simulink model "csu_gmb_gimbal_motor_actuator_diag"  (R2015b)
settings: Solver=VariableStepAuto  StartTime=0.0  StopTime=10.0  RelTol=1e-3
values from neighbouring files (symbols this model uses):
  Bm = gim_motor_Bm    [csu_gmb_motor_prep.m]
  Jm = gim_motor_Jm    [csu_gmb_motor_prep.m]
  Ke = gim_motor_Ke    [csu_gmb_motor_prep.m]
  Kl = gim_motor_Kl    [csu_gmb_motor_prep.m]
  Kt = gim_motor_Kt    [csu_gmb_motor_prep.m]
  Lm = gim_motor_Lm    [csu_gmb_motor_prep.m]
  nb = gim_motor_nb    [csu_gmb_motor_prep.m]
  Rm = gim_motor_Rm    [csu_gmb_motor_prep.m]
undefined symbols (not defined in the file or in its folder): DiscIntNeverNeededParam
settings Model: Creator=jimkaidy  LastModifiedBy=jimkaidy

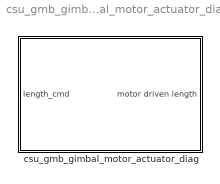
== system csu_gmb_gimbal_motor_actuator_diag ==
  csu_gmb_gimbal_motor_actuator_diag : Subsystem

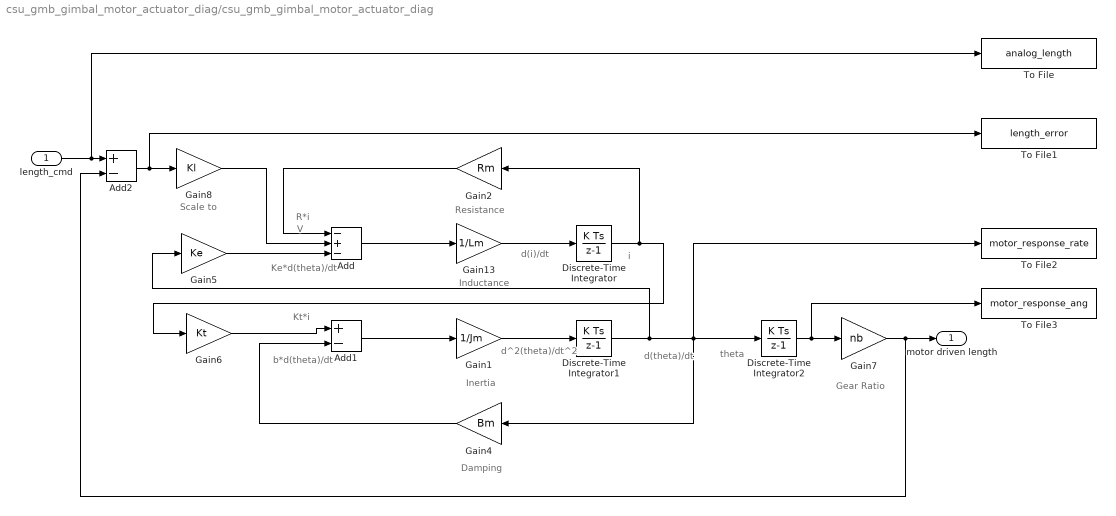
== system csu_gmb_gimbal_motor_actuator_diag/csu_gmb_gimbal_motor_actuator_diag ==
  note: Scale to
  note: theta
  note: d^2(theta)/dt^2
  note: b*d(theta)/dt
  note: Kt*i
  note: d(theta)/dt
  note: Ke*d(theta)/dt
  note: V
  note: R*i
  note: i
  note: d(i)/dt
  note: Gear Ratio
  note: Resistance
  note: Damping
  note: Inertia
  note: Inductance
  length_cmd : Inport
  Add : Sum  Inputs=-+-
  Add1 : Sum  Inputs=+-
  Add2 : Sum  Inputs=+-
  Discrete-Time Integrator : DiscreteIntegrator  InitialConditionSetting=State (most efficient)  SampleTime=-1  ICPrevOutput=DiscIntNeverNeededParam  ICPrevScaledInput=DiscIntNeverNeededParam
  Discrete-Time Integrator1 : DiscreteIntegrator  InitialConditionSetting=State (most efficient)  SampleTime=-1  ICPrevOutput=DiscIntNeverNeededParam  ICPrevScaledInput=DiscIntNeverNeededParam
  Discrete-Time Integrator2 : DiscreteIntegrator  InitialConditionSetting=State (most efficient)  SampleTime=-1  ICPrevOutput=DiscIntNeverNeededParam  ICPrevScaledInput=DiscIntNeverNeededParam
  Gain1 : Gain  Gain=1/Jm
  Gain13 : Gain  Gain=1/Lm
  Gain2 : Gain  Gain=Rm
  Gain4 : Gain  Gain=Bm
  Gain5 : Gain  Gain=Ke
  Gain6 : Gain  Gain=Kt
  Gain7 : Gain  Gain=nb
  Gain8 : Gain  Gain=Kl
  To File : ToFile  Filename=analog_length  MatrixName=analog_length  SaveFormat=Timeseries
  To File1 : ToFile  Filename=length_error  MatrixName=length_error  SaveFormat=Timeseries
  To File2 : ToFile  Filename=motor_response_rate  MatrixName=motor_response_rate  SaveFormat=Timeseries
  To File3 : ToFile  Filename=motor_response_ang  MatrixName=motor_response_ang  SaveFormat=Timeseries
  motor driven length : Outport
  wires:
  length_cmd/1 -> To File/1, Add2/1
  Gain13/1 -> Discrete-Time Integrator/1
  Gain1/1 -> Discrete-Time Integrator1/1
  Gain5/1 -> Add/3
  Gain4/1 -> Add1/2
  Gain2/1 -> Add/1
  Gain6/1 -> Add1/1
  Discrete-Time Integrator/1 -> Gain2/1, Gain6/1
  Gain8/1 -> Add/2
  Add/1 -> Gain13/1
  Add1/1 -> Gain1/1
  Discrete-Time Integrator1/1 -> Gain5/1, To File2/1, Gain4/1, Discrete-Time Integrator2/1
  Add2/1 -> To File1/1, Gain8/1
  Discrete-Time Integrator2/1 -> To File3/1, Gain7/1
  Gain7/1 -> Add2/2, motor driven length/1
